simulink model "STRbase_Final_r2022a_final"  (R2022a)
settings: Solver=VariableStepAuto  StartTime=0.0  StopTime=500  RelTol=1e-3
settings Model: Creator=user  LastModifiedBy=user
settings DebuggingCC: UnderSpecifiedDimensionMsg=warning

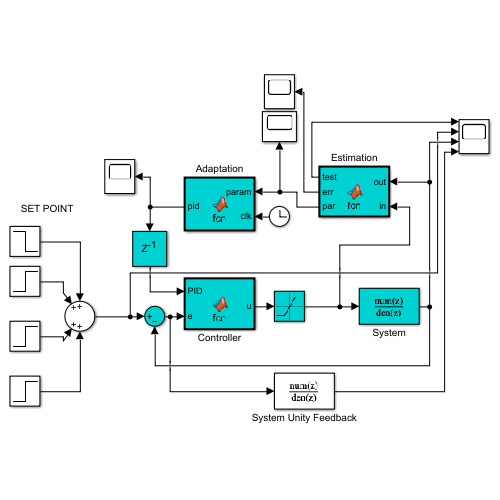
[thumbnail: Simulink's stored preview of the top-level diagram]
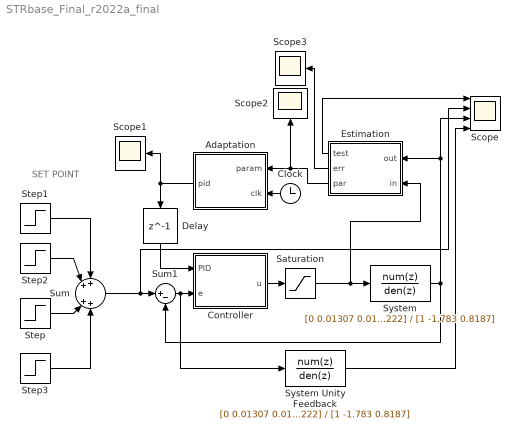
== system STRbase_Final_r2022a_final ==
  note: SET POINT
  Adaptation : MATLAB Function  TreatAsAtomicUnit=on
  Clock : Clock
  Controller : MATLAB Function  TreatAsAtomicUnit=on
  Delay : Delay  DelayLength=1
  Estimation : MATLAB Function  TreatAsAtomicUnit=on
  Saturation : Saturate  UpperLimit=20  LowerLimit=-20
  Scope : Scope  NumInputPorts=4
  Scope1 : Scope
  Scope2 : Scope
  Scope3 : Scope
  Step : Step  Time=50  After=9  SampleTime=0
  Step1 : Step  Time=80  After=-2  SampleTime=0
  Step2 : Step  Time=100  SampleTime=0
  Step3 : Step  Time=160  After=6  SampleTime=0
  Sum : Sum  Inputs=++||++
  Sum1 : Sum  Inputs=|+-
  System : DiscreteTransferFcn  Numerator=[0 0.01307 0.01222]  Denominator=[1 -1.783 0.8187]  InitialStates=10  SampleTime=0.5
  System Unity Feedback : DiscreteTransferFcn  Numerator=[0 0.01307 0.01222]  Denominator=[1 -1.783 0.8187]  InitialStates=10  SampleTime=0.5
  wires:
  System/1 -> Sum1/2, Scope/3, Estimation/1(out)
  Estimation/1(test) -> Scope/1
  Step/1 -> Sum/3
  Adaptation/1(pid) -> Delay/1, Scope1/1
  Delay/1 -> Controller/1(PID)
  Clock/1 -> Adaptation/2(clk)
  Controller/1(u) -> Saturation/1
  Saturation/1 -> Estimation/2(in), System/1
  Step2/1 -> Sum/2
  Sum/1 -> Scope/2, Sum1/1
  Sum1/1 -> System Unity Feedback/1, Controller/2(e)
  Estimation/2(err) -> Scope3/1
  Step3/1 -> Sum/4
  System Unity Feedback/1 -> Scope/4
  Estimation/3(par) -> Scope2/1, Adaptation/1(param)
  Step1/1 -> Sum/1

== matlab function STRbase_Final_r2022a_final/Controller ==
  data: PID input; u output size=1; e input
function u   = fcn(PID, e)
Kp = 1;
Ki = 0;
Kd = 0;
ts=0.5;
persistent prev_error int_error

if isempty(prev_error)
    prev_error=0;
end

if isempty(int_error)
    int_error=0;
end

    %[kp, ki, kd] = PID
    int_error = int_error + e;
    derivative = e - prev_error;

    %Kp = 0.2*Kp+0.8*(PID(1)-Kp)*PID(1)/Kp;
    %Ki = 0.2*Ki+0.8*PID(2);
    %Kd = 0.2*Kd+0.8*PID(3);

    %Kp = 0.2*Kp+0.8*KpA;
    %Ki = 0.2*Ki+0.8*KiA;
    %Kd = 0.2*Kd+0.8*KdA;
    Kp=PID(1);
    Ki=PID(2);
    Kd=PID(3);

    u = Kp * e + Ki * int_error + Kd * derivative;
    %u = Kp * e + Ki * int_error + Kd * diff(e);
u = u;

end

== matlab function STRbase_Final_r2022a_final/Estimation ==
  data: out input; in input; test output; err output; par output
function [test,err,par] = fcn(out,in)
%untuk sekarang dibatasin cmn khusus identifikasi dengan orde 2
m=2;
n=2;
lbd=0.97;
persistent ind outd P W 

if isempty(P)
    P=eye(m+n);
end

if isempty(W)
    W=zeros(m+n,1);    
end

if isempty(ind);
    ind=zeros(m,1);
end

if isempty(outd)
    outd=zeros(n,1);
end

%RLS nya
%matrix parameter w mengikuti bentuk x
%x = [y(k-1) y(k-2) u(k-1) u(k-2)]'

%param w kalau di transfer function penjelasan ada di function block
%Adaptation
    x = [outd;ind];
    phi = P*x;
    g = phi/(lbd+x'*phi);
    o = W;
    y= o'*x;
    e = out-y;
    W= W+g*e*1;
    P = (P-g*x'*P)/lbd;

outd=[out;outd(1:1:end-1,:)];
ind=[in;ind(1:1:end-1,:)];

par=W;

%test output variabel apa aja, default nya output RLS yaitu y
test=y;
err=e;
end

== matlab function STRbase_Final_r2022a_final/Adaptation ==
  data: param input; pid output; clk input
function pid  = fcn(param,clk)
%parameternya ini dibagi jadi dua part
%anggap sistem diskrit dengan 
%NUM = [0 b1 b2]
%DEN = [1 a1 a2]
%param=[-a1 -a2 b1 b2]

%param(1) itu koef -y(k-1) atau klo di DEN itu -a1 
%param(2) itu koef -y(k-2) atau klo di DEN itu -a2

%param(3) itu koef u(k-1) atau klo di DEN itu b1 
%param(4) itu koef u(k-2) atau klo di DEN itu b2
persistent PID
if isempty(PID)
    PID=[1 0 0];
end
coder.extrinsic("tf","pidtune","piddata")

if mod(clk,10)==0
    a1 = -param(1);
    a2 = -param(2);
    b1 = param(3);
    b2 = param(4);
    
    num = [0 b1 b2];
    den = [1 a1 a2];
    Tf = tf(num,den,0.5);
    
    % [kc,pm,wc,wm] = margin(Tf)
    % pu = 2*pi/wc
    
    %PID Parameter
    
    [C] = pidtune(Tf, 'PID');
    [kp, ki, kd] = piddata(C);
    
    % kp = kc*0.59;
    % ti = pu*0.5;
    % td = pu*0.12;
    % ki = kp/ti;
    % kd = kp*td;
    
    PID = [kp ki kd];
end
pid=PID;
end
